simulink model "tempreture_2_5"  (R2021a)
settings: Solver=VariableStepAuto  StartTime=0.0  StopTime=60  RelTol=1e-3
libraries: simulink x3
settings Model: Creator=yasso  LastModifiedBy=yasso

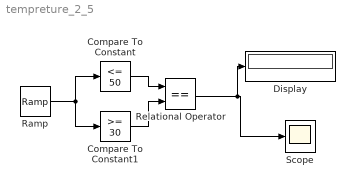
== system tempreture_2_5 ==
  Compare To Constant : simulink/Logic and Bit Operations/Compare To Constant  relop=<=  const=50  OutDataTypeStr=boolean
  Compare To Constant1 : simulink/Logic and Bit Operations/Compare To Constant  relop=>=  const=30  OutDataTypeStr=boolean
  Display : Display
  Ramp : simulink/Sources/Ramp  slope=1  start=0  InitialOutput=0
  Relational Operator : RelationalOperator  Operator===  OutDataTypeStr=boolean  RndMeth=Simplest
  Scope : Scope
  wires:
  Ramp/1 -> Compare To Constant1/1, Compare To Constant/1
  Compare To Constant1/1 -> Relational Operator/2
  Compare To Constant/1 -> Relational Operator/1
  Relational Operator/1 -> Display/1, Scope/1
